simulink model "preSPEA"  (R2015a)
settings: Solver=ode45  StartTime=0.0  StopTime=10.0  RelTol=1e-3
values from neighbouring files (symbols this model uses):
  b_L = 1e-5    (= 1e-05)    [parameters.m]
  b_m = 1e-5    (= 1e-05)    [parameters.m]
  g = 9.81    [parameters.m]
  J_L = J_ts + J_hubf + J_hub + J_shaft + J_arm    (= 0.04931437)    [parameters.m]
  J_m = J_motor    (= 0.0002832)    [parameters.m]
  k_p = 1    [parameters.m]
  k_s = i    [multi_pass.m]    (also in parameters.m = 124)
  l = 0.16    [parameters.m]
  m = 1.9113    [parameters.m]
  tau_max = 5    [parameters.m]
  theta_c = 0    [parameters.m]
  theta_L0 = deg2rad(0)    [parameters.m]
  theta_m0 = deg2rad(0)    [parameters.m]
settings Model: Creator=Nathan  LastModifiedBy=Nathan

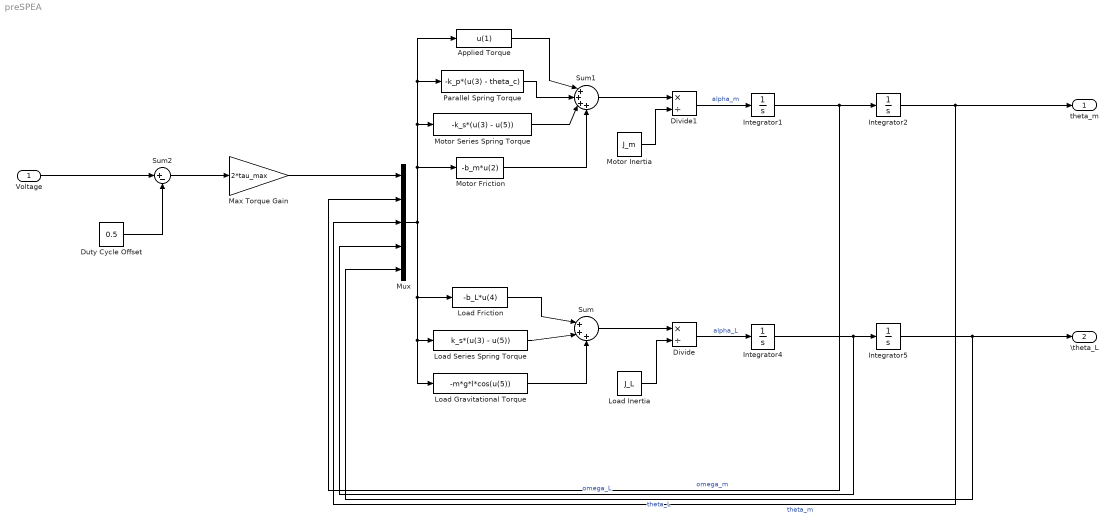
== system preSPEA ==
  Voltage : Inport
  Applied Torque : Fcn  Expr=u(1)
  Divide : Product  Inputs=*/
  Divide1 : Product  Inputs=*/
  Duty Cycle Offset : Constant  Value=0.5
  Integrator1 : Integrator
  Integrator2 : Integrator  InitialCondition=theta_m0
  Integrator4 : Integrator
  Integrator5 : Integrator  InitialCondition=theta_L0
  Load Friction : Fcn  Expr=-b_L*u(4)
  Load Gravitational Torque : Fcn  Expr=-m*g*l*cos(u(5))
  Load Inertia : Constant  Value=J_L
  Load Series Spring Torque : Fcn  Expr=k_s*(u(3) - u(5))
  Max Torque Gain : Gain  Gain=2*tau_max
  Motor Friction : Fcn  Expr=-b_m*u(2)
  Motor Inertia : Constant  Value=J_m
  Motor Series Spring Torque : Fcn  Expr=-k_s*(u(3) - u(5))
  Mux : Mux  Inputs=5
  Parallel Spring Torque : Fcn  Expr=-k_p*(u(3) - theta_c)
  Sum : Sum  Inputs=|+++
  Sum1 : Sum  Inputs=|++++
  Sum2 : Sum  Inputs=|+-
  "theta_m " : Outport
  \theta_L : Outport  Port=2
  wires:
  Divide/1 -> Integrator4/1  "alpha_L"
  Integrator5/1 -> \theta_L/1, Mux/5  "theta_L"
  Mux/1 -> Load Friction/1, Load Series Spring Torque/1, Load Gravitational Torque/1, Motor Friction/1, Motor Series Spring Torque/1, Applied Torque/1, Parallel Spring Torque/1
  Load Inertia/1 -> Divide/2
  Sum/1 -> Divide/1
  Load Friction/1 -> Sum/1
  Load Series Spring Torque/1 -> Sum/2
  Load Gravitational Torque/1 -> Sum/3
  Integrator4/1 -> Integrator5/1, Mux/4  "omega_L"
  Integrator1/1 -> Integrator2/1, Mux/2  "omega_m"
  Integrator2/1 -> "theta_m "/1, Mux/3  "theta_m"
  Motor Inertia/1 -> Divide1/2
  Divide1/1 -> Integrator1/1  "alpha_m"
  Sum1/1 -> Divide1/1
  Applied Torque/1 -> Sum1/1
  Parallel Spring Torque/1 -> Sum1/2
  Motor Series Spring Torque/1 -> Sum1/3
  Motor Friction/1 -> Sum1/4
  Voltage/1 -> Sum2/1
  Duty Cycle Offset/1 -> Sum2/2
  Sum2/1 -> Max Torque Gain/1
  Max Torque Gain/1 -> Mux/1
